simulink model "drive"  (R2024b)
settings: Solver=VariableStepAuto  StartTime=0.0  StopTime=10.0  RelTol=1e-3
InitFcn:
  | driveIni
values from neighbouring files (symbols this model uses):
  kr = Xm/Xr    [driveIni.m]
  omegaM_ref = 0.9    [driveIni.m]
  PWMrat = 39    [driveIni.m]
  Rs = Rs_SI/Zb    [driveIni.m]
  Rsigma = Rs + kr^2 * Rr    [driveIni.m]
  sigma = 1 - (Xm^2 / (Xr * Xs))    [driveIni.m]
  tauR = Xr / Rr    [driveIni.m]
  tauS = Xr * D / (Rs * Xr^2 + Rr * Xm^2)    [driveIni.m]
  TL_ini = 0.3    [driveIni.m]
  Ts = 1e-6    (= 1e-06)    [driveIni.m]
  Vdc = Vdc_nom_SI/Vb    [driveIni.m]
  Vf = 1    [driveIni.m]
  w_b = wb    [driveIni.m]
  Xm = wb*Lm_SI/Zb    [driveIni.m]
  Xr = Xlr + Xm    [driveIni.m]
  Xs = Xls + Xm    [driveIni.m]
undefined symbols (not defined in the file or in its folder): J
libraries: matrix_library x1
settings Model: Creator=PetrosK  LastModifiedBy=horak
settings DebuggingCC: UnderspecifiedInitializationDetection=Classic  MergeDetectMultiDrivingBlocksExec=none
settings ModelReferenceCC: PropagateSignalLabelsOutOfModel=off

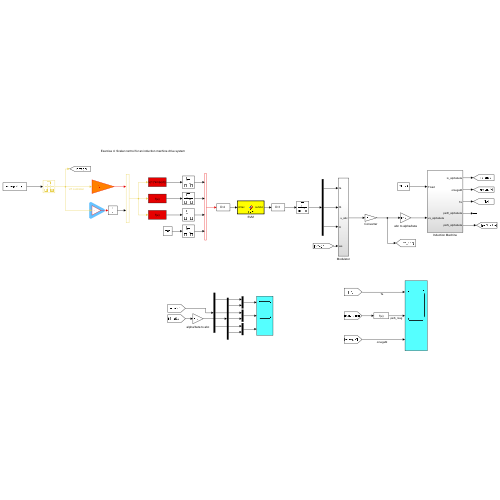
[thumbnail: Simulink's stored preview of the top-level diagram]
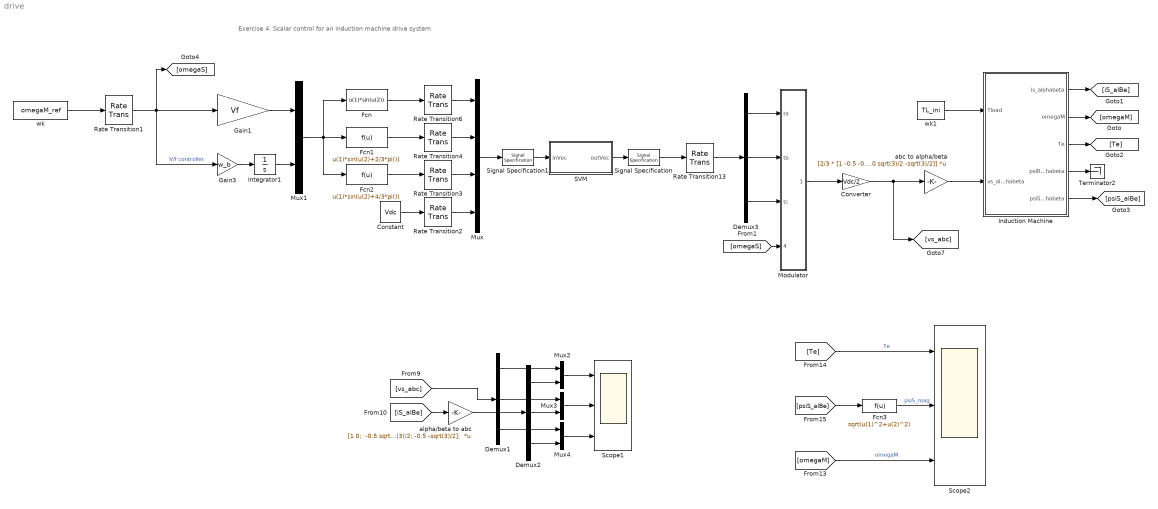
== system drive ==
  note: Exercise 4: Scalar control for an induction machine drive system
  Constant : Constant  Value=Vdc  VectorParams1D=off
  Converter : Gain  Gain=Vdc/2  SaturateOnIntegerOverflow=on  OutDataTypeStr=Inherit: Same as input  ParamDataTypeStr=Inherit: Same as input
  Demux1 : Demux  Outputs=3
  Demux2 : Demux  Outputs=3
  Demux3 : Demux  Outputs=3
  Fcn : Fcn  Expr=u(1)*sin(u(2))
  Fcn1 : Fcn  Expr=u(1)*sin(u(2)+2/3*pi())
  Fcn2 : Fcn  Expr=u(1)*sin(u(2)+4/3*pi())
  Fcn3 : Fcn  Expr=sqrt(u(1)^2+u(2)^2)
  Gain1 : Gain  Gain=Vf
  Gain3 : Gain  Gain=w_b
  Induction Machine : Subsystem
  Integrator1 : Integrator
  Modulator : Subsystem
  Mux : Mux
  Mux{1..4} (4 alike) : Mux  Inputs=2
  Rate Transition1 : RateTransition  Deterministic=off  OutPortSampleTime=Ts
  Rate Transition13 : RateTransition  Deterministic=off  OutPortSampleTime=Ts
  Rate Transition{2..4,6} (4 alike) : RateTransition  Deterministic=off  OutPortSampleTime=Tc
  SVM : MATLAB Function  TreatAsAtomicUnit=on
  Scope1 : Scope  NumInputPorts=3
  Scope2 : Scope  NumInputPorts=3
  Signal Specification : SignalSpecification  Dimensions=3
  Signal Specification1 : SignalSpecification  Dimensions=4
  Terminator2 : Terminator
  abc to alpha/beta : Gain  Gain=[2/3 * [1 -0.5 -0.5;0 sqrt(3)/2 -sqrt(3)/2]]  Multiplication=Matrix(K*u)  SaturateOnIntegerOverflow=on  OutDataTypeStr=Inherit: Same as input  ParamDataTypeStr=Inherit: Same as input
  alpha/beta to abc : Gain  Gain="[1 0;  -0.5 sqrt(3)/2; -0.5 -sqrt(3)/2];"  Multiplication=Matrix(K*u)  SaturateOnIntegerOverflow=on  OutDataTypeStr=Inherit: Same as input  ParamDataTypeStr=Inherit: Same as input
  wk : Constant  Value=omegaM_ref  VectorParams1D=off
  wk1 : Constant  Value=TL_ini  VectorParams1D=off
  wires:
  abc to alpha/beta/1 -> Induction Machine/2(vs_alphabeta)
  Induction Machine/1(is_alphabeta) -> [iS_alBe]
  Induction Machine/4(psiR_alphabeta) -> Terminator2/1
  Induction Machine/3(Te) -> [Te]
  Induction Machine/5(psiS_alphabeta) -> [psiS_alBe]
  Induction Machine/2(omegaM) -> [omegaM]
  SVM/1(outVec) -> Signal Specification/1
  Demux3/2 -> Modulator/2(tb)
  Demux3/3 -> Modulator/3(tc)
  Demux3/1 -> Modulator/1(ta)
  Constant/1 -> Rate Transition2/1
  Rate Transition13/1 -> Demux3/1
  Rate Transition1/1 -> Gain1/1, Gain3/1, [omegaS]  "V/f controller"
  [omegaM] -> Scope2/3  "omegaM"
  Fcn3/1 -> Scope2/2  "psiS_mag"
  [psiS_alBe] -> Fcn3/1
  [Te] -> Scope2/1  "Te"
  Mux2/1 -> Scope1/1
  Mux3/1 -> Scope1/2
  Mux4/1 -> Scope1/3
  Demux1/1 -> Mux2/1
  alpha/beta to abc/1 -> Demux2/1
  Demux2/1 -> Mux2/2
  [iS_alBe] -> alpha/beta to abc/1
  Demux1/2 -> Mux3/1
  Demux1/3 -> Mux4/1
  Demux2/2 -> Mux3/2
  Demux2/3 -> Mux4/2
  [vs_abc] -> Demux1/1
  Modulator/1(u_abc) -> Converter/1
  Converter/1 -> [vs_abc], abc to alpha/beta/1
  Signal Specification1/1 -> SVM/1(inVec)
  Signal Specification/1 -> Rate Transition13/1
  Mux/1 -> Signal Specification1/1
  Rate Transition2/1 -> Mux/4
  Rate Transition3/1 -> Mux/3
  Rate Transition4/1 -> Mux/2
  Rate Transition6/1 -> Mux/1
  Fcn/1 -> Rate Transition6/1
  Fcn1/1 -> Rate Transition4/1
  Fcn2/1 -> Rate Transition3/1
  Mux1/1 -> Fcn2/1, Fcn/1, Fcn1/1
  [omegaS] -> Modulator/4(ws)
  Gain1/1 -> Mux1/1
  Gain3/1 -> Integrator1/1
  Integrator1/1 -> Mux1/2
  wk/1 -> Rate Transition1/1
  wk1/1 -> Induction Machine/1(Tload)

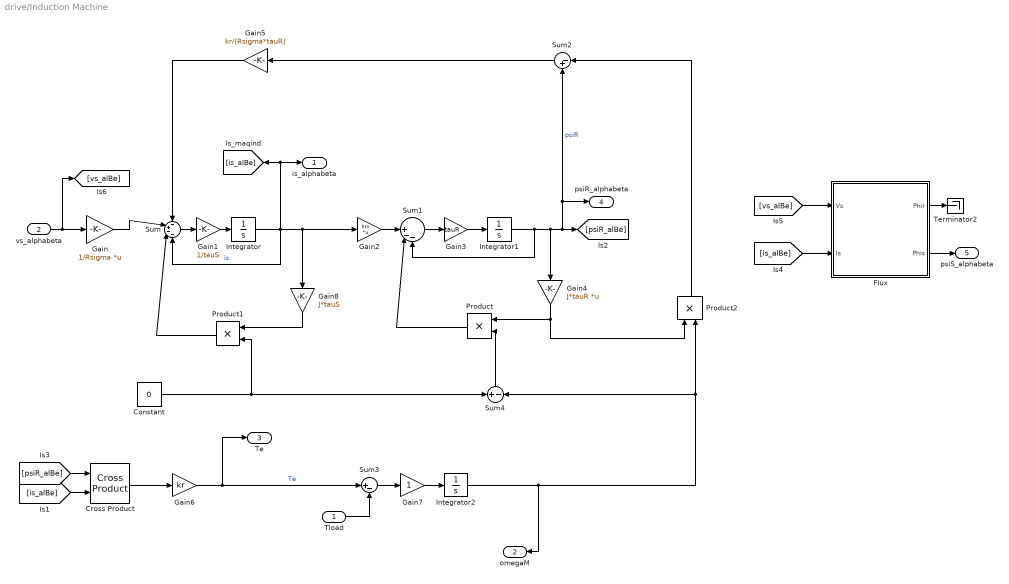
== system drive/Induction Machine ==
  Tload : Inport
  vs_alphabeta : Inport  Port=2
  Constant : Constant  Value=0
  Cross Product : matrix_library/Cross Product
  Flux : Subsystem
  Gain : Gain  Gain=1/Rsigma  Multiplication=Matrix(K*u)
  Gain1 : Gain  Gain=1/tauS
  Gain2 : Gain  Gain=Xm  Multiplication=Matrix(K*u)
  Gain3 : Gain  Gain=tauR
  Gain4 : Gain  Gain=J*tauR  Multiplication=Matrix(K*u)
  Gain5 : Gain  Gain=kr/(Rsigma*tauR)
  Gain6 : Gain  Gain=kr
  Gain7 : Gain
  Gain8 : Gain  Gain=J*tauS
  Integrator : Integrator
  Integrator1 : Integrator
  Integrator2 : Integrator
  Product : Product
  Product1 : Product
  Product2 : Product
  Sum : Sum  Inputs=-+--
  Sum1 : Sum  Inputs=||+--
  Sum2 : Sum  Inputs=|-+
  Sum3 : Sum  Inputs=|+-
  Sum4 : Sum  Inputs=+|-
  Terminator2 : Terminator
  is_alphabeta : Outport
  omegaM : Outport  Port=2
  Te : Outport  Port=3
  psiR_alphabeta : Outport  Port=4
  psiS_alphabeta : Outport  Port=5
  wires:
  [is_alBe] -> Cross Product/2
  [psiR_alBe] -> Cross Product/1
  vs_alphabeta/1 -> Gain/1, [vs_alBe]
  Flux/2(Phis) -> psiS_alphabeta/1
  Flux/1(Phir) -> Terminator2/1
  [is_alBe] -> Flux/2(Is)
  [vs_alBe] -> Flux/1(Vs)
  Integrator/1 -> Gain2/1, Gain8/1, is_alphabeta/1, [is_alBe], Sum/4  "is"
  Gain6/1 -> Te/1, Sum3/1  "Te"
  Integrator2/1 -> Sum4/2, Product2/2, omegaM/1
  Gain/1 -> Sum/2
  Sum/1 -> Gain1/1
  Gain1/1 -> Integrator/1
  Gain2/1 -> Sum1/1
  Sum1/1 -> Gain3/1
  Gain3/1 -> Integrator1/1
  Integrator1/1 -> [psiR_alBe], psiR_alphabeta/1, Sum2/2, Gain4/1, Sum1/3  "psiR"
  Gain4/1 -> Product2/1, Product/1
  Product/1 -> Sum1/2
  Gain5/1 -> Sum/1
  Sum2/1 -> Gain5/1
  Cross Product/1 -> Gain6/1
  Tload/1 -> Sum3/2
  Gain7/1 -> Integrator2/1
  Sum3/1 -> Gain7/1
  Sum4/1 -> Product/2
  Gain8/1 -> Product1/1
  Product1/1 -> Sum/3
  Product2/1 -> Sum2/1
  Constant/1 -> Sum4/1, Product1/2

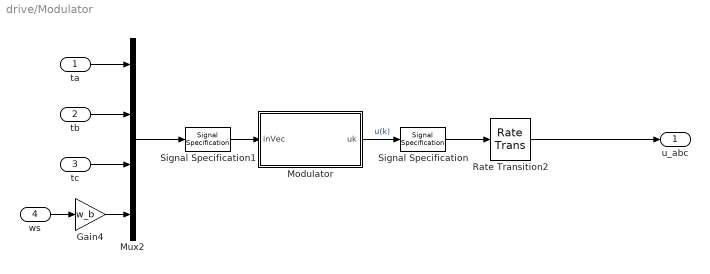
== system drive/Modulator ==
  ta : Inport
  tb : Inport  Port=2
  tc : Inport  Port=3
  ws : Inport  Port=4
  Gain4 : Gain  Gain=w_b
  Modulator : MATLAB Function  TreatAsAtomicUnit=on
  Mux2 : Mux
  Rate Transition2 : RateTransition  OutPortSampleTime=Ts
  Signal Specification : SignalSpecification  Dimensions=3
  Signal Specification1 : SignalSpecification  Dimensions=4
  u_abc : Outport
  wires:
  ta/1 -> Mux2/1
  tb/1 -> Mux2/2
  tc/1 -> Mux2/3
  Modulator/1(uk) -> Signal Specification/1  "u(k)"
  Signal Specification/1 -> Rate Transition2/1
  Rate Transition2/1 -> u_abc/1
  Mux2/1 -> Signal Specification1/1
  ws/1 -> Gain4/1
  Signal Specification1/1 -> Modulator/1(inVec)
  Gain4/1 -> Mux2/4

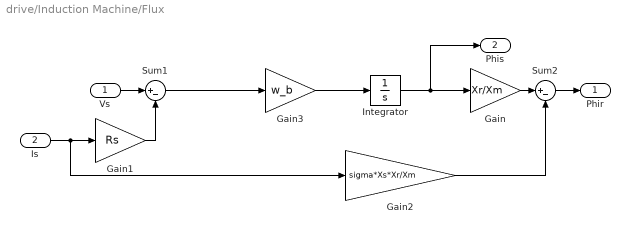
== system drive/Induction Machine/Flux ==
  Vs : Inport
  Is : Inport  Port=2
  Gain : Gain  Gain=Xr/Xm
  Gain1 : Gain  Gain=Rs
  Gain2 : Gain  Gain=sigma*Xs*Xr/Xm
  Gain3 : Gain  Gain=w_b
  Integrator : Integrator
  Sum1 : Sum  Inputs=|+-
  Sum2 : Sum  Inputs=|+-
  Phir : Outport
  Phis : Outport  Port=2
  wires:
  Is/1 -> Gain1/1, Gain2/1
  Gain1/1 -> Sum1/2
  Sum1/1 -> Gain3/1
  Integrator/1 -> Gain/1, Phis/1
  Gain/1 -> Sum2/1
  Gain2/1 -> Sum2/2
  Vs/1 -> Sum1/1
  Sum2/1 -> Phir/1
  Gain3/1 -> Integrator/1

== matlab function drive/Modulator/Modulator ==
  data: inVec input; uk output; PWMrat parameter; Ts parameter
function uk = modulator(inVec, PWMrat, Ts)

% generation of switching signals for a three-phase two-level inverter
%
% Control of Electrical Drive Systems, TAU, Tampere
% Petros Karamanakos, September 2025

persistent kk carrier t 

% interface
t_a = 2 * inVec(1) - 1; % modulating signal of phase a in [-1, 1]
t_b = 2 * inVec(2) - 1;	% modulating signal of phase b in [-1, 1]
t_c = 2 * inVec(3) - 1; % modulating signal of phase c in [-1, 1]
w  = inVec(4);          % angular speed [pu]

t = [t_a; t_b; t_c];

if isempty(kk)
    kk = 1;
    carrier = 0;
    t_smpl = t;
end

% fundamental frequency/period
f_1 = w/(2 * pi);
T_1 = 1/f_1;

% period of carrier
TsPWM = T_1/PWMrat;

%% build the carrier 

if kk * Ts < TsPWM
    triangleStep = 4*Ts/TsPWM;
    if kk*Ts <= TsPWM/4
        carrier = carrier - triangleStep;
    elseif kk*Ts > TsPWM/4 &&  kk*Ts <= 3*TsPWM/4
        carrier = carrier + triangleStep;
    else
        carrier = carrier - triangleStep;
    end
else 
    kk = 0;
    carrier = 0;
end
kk = kk + 1;

%% generate the switching signals 

if t(1) >= carrier
    u_a = 1;
else
    u_a = -1;
end

if t(2) >= carrier
    u_b = 1;
else
    u_b = -1;
end

if t(3) >= carrier
    u_c = 1;
else
    u_c = -1;
end

%% output signal

uk = [u_a; u_b; u_c];   % three-phase switch position

return

== matlab function drive/SVM ==
  data: inVec input; outVec output
function outVec = SVM(inVec)

% SVM for a three-phase two-level inverter
%
% Control of Electrical Drive Systems, TAU, Tampere
% Petros Karamanakos, September 2025

v_a = inVec(1);
v_b = inVec(2);
v_c = inVec(3);
Vdc = inVec(4);

v_abc = [v_a; v_b; v_c];

% reduced Clarke transformation
K = 2/3 * [1 -0.5 -0.5;           	% abc -> alpha/beta
           0 sqrt(3)/2 -sqrt(3)/2];     
           
% modulating signal
v_ab0 = 2/Vdc * K * v_abc; 

% alpha/beta components
v_alpha = v_ab0(1);
v_beta = v_ab0(2);

% modulating signal in alpha/beta
m_albe = complex(v_alpha, v_beta); 
m_ref = abs(m_albe);
m_angl = angle(m_albe);
V = 4/3;

% sector of reference vector 
Sector = ceil(m_angl / (pi/3));
if Sector < 1
    Sector = Sector + 6;
end

% ta, tb, t0 based on Cramer's rule
D = det([V, V * cos(pi/3); V * cos(pi/3), V]);  
if Sector < 4
    Dta = det([m_ref * cos(m_angl - (Sector - 1) * pi/3)	V * cos(pi/3); 
               m_ref * cos(Sector * pi/3 - m_angl)          V]);       
    Dtb = det([     V           m_ref * cos(m_angl - (Sector - 1) * pi/3); 
               V * cos(pi/3)    m_ref * cos(Sector * pi/3 - m_angl)]);
else
    Dta = det([m_ref * cos(m_angl - (Sector - 7) * pi/3)    V * cos(pi/3);
               m_ref * cos((Sector - 6) * pi/3 - m_angl)    V]);       
    Dtb = det([     V           m_ref * cos(m_angl - (Sector - 7) * pi/3);
               V * cos(pi/3)    m_ref * cos((Sector - 6) *pi/3 - m_angl)]);
end    

ta = Dta / D; % application time of voltage vector v_i
tb = Dtb / D; % application time of voltage vector v_j
t0 = 1 - ta - tb; % application time of zero vectors

% calculation of application times based on sectors
if Sector == 1
    t1 = ta + tb + t0/2;
    t3 = tb + t0/2;
    t5 = t0/2;
elseif Sector == 2
    t1 = ta + t0/2;
    t3 = ta + tb + t0/2;
    t5 = t0/2;
elseif Sector == 3
    t1 = t0/2;
    t3 = ta + tb + t0/2;
    t5 = tb + t0/2;
elseif Sector == 4
    t1 = t0/2;
    t3 = ta + t0/2;
    t5 = ta + tb + t0/2;
elseif Sector==5
    t1 = tb + t0/2;
    t3 = t0/2;
    t5 = ta + tb + t0/2;
else
    t1 = ta + tb + t0/2;
    t3 = t0/2;
    t5 = ta + t0/2;
end

%% switching times for the three upper switches

outVec = [t1; t3; t5];

return
